simulink model "Test14Dof"  (R2024a)
settings: Solver=ode4  StartTime=0.0  StopTime=10.0  FixedStep=0.001  RelTol=1e-3
values from neighbouring files (symbols this model uses):
  EnvGrvty = 9.81    [Par.m]
  PlntBattChrgMax = 4.493    [Par.m]
  PlntBattNumCellSer = 96    [Par.m]
  PlntBattOpenCirctVolt = [3.17242 3.17242 3.17242 3.17242 3.17242 3.17242 3.17242;3.18272 3.18272 3.18272 3.18272 3.18272 3.18272 3.18272;3.19302 3.19302 3.19302 3.19302 3.19302 3.19302 3.19302;3.20331 3.20331 3.20331 3.20331 3.20331 3.20331 3.20331;3.21361 3.21361 3.21361 3.21361 3.21361 3.21361 3.21361;3.22391 3.22391 3.22391 3.22391 3.22391 3.22391 3.22391;3.23421 3.23421 3.23421 3.23421 3.23421 3.23421 3.23421;3.24451 ...(+5187 chars)    [Par.m]
  PlntBattSocInit = 0.6    [Par.m]
  PlntBattTempBpt = [-40 -30 -20 0 23 45 60]    [Par.m]
  PlntBattTempInitDegC = 25    [Par.m]
  PlntBattVoltSocBpt = [0 0.01 0.02 0.03 0.04 0.05 0.06 0.07 0.08 0.09 0.1 0.11 0.12 0.13 0.14 0.15 0.16 0.17 0.18 0.19 0.2 0.21 0.22 0.23 0.24 0.25 0.26 0.27 0.28 0.29 0.3 0.31 0.32 0.33 0.34 0.35 0.36 0.37 0.38 0.39 0.4 0.41 0.42 0.43 0.44 0.45 0.46 0.47 0.48 0.49 0.5 0.51 0.52 0.53 0.54 0.55 0.56 0.57 0.58 0.59 0.6 0.61 0.62 0.63 0.64 0.65 0.66 0.67 0.68 0.69 0.7 0.71 0.72 0.73 0.74 0.75 0.76 0.77 0.78 0.79 0.8 0.81  ...(+91 chars)    [Par.m]
  PlntDCDCVoltInit = 650    [Par.m]
  PlntDriveshftDamp = 100    [Par.m]
  PlntDriveshftStiff = 500    [Par.m]
  PlntEM1RotDamp = 0.001    [Par.m]
  PlntEM1RotInertia = 0.01    [Par.m]
  PlntEM2RotDamp = 0.001    [Par.m]
  PlntEM2RotInertia = 0.01    [Par.m]
  PlntEM3RotDamp = 0.001    [Par.m]
  PlntEM3RotInertia = 0.01    [Par.m]
  PlntEM4RotDamp = 0.001    [Par.m]
  PlntEM4RotInertia = 0.01    [Par.m]
  PlntEMWhlGearRatioFL = 11.04    [Par.m]
  PlntEMWhlGearRatioFR = 11.04    [Par.m]
  PlntEMWhlGearRatioRL = 11.04    [Par.m]
  PlntEMWhlGearRatioRR = 11.04    [Par.m]
  PlntSteerGearRatio = 52.025    [Par.m]
  PlntVehCGHgtAxl = 0.375    [Par.m]
  PlntVehDstCGFrntAxl = 1.61    [Par.m]
  PlntVehDstCGRearAxl = 1.39    [Par.m]
  PlntVehFrntUnsprgMass = 100    [Par.m]
  PlntVehInitLatPos = 0    [Par.m]
  PlntVehInitLatVel = 0    [Par.m]
  PlntVehInitLongPos = 0    [Par.m]
  PlntVehInitLongVel = 0    [Par.m]
  PlntVehInitPitchAng = 0    [Par.m]
  PlntVehInitPitchRate = 0    [Par.m]
  PlntVehInitRollAng = 0    [Par.m]
  PlntVehInitRollRate = 0    [Par.m]
  PlntVehInitVertPos = 0    [Par.m]
  PlntVehInitVertVel = 0    [Par.m]
  PlntVehInitYawAng = 0    [Par.m]
  PlntVehInitYawRate = 0    [Par.m]
  PlntVehMass = 2497    [Par.m]
  PlntVehPitchMomentInertia = 1922.7    [Par.m]
  PlntVehRearUnsprgMass = 100    [Par.m]
  PlntVehRollMomentInertia = 432.33333333333331    (= 432.333333333)    [Par.m]
  PlntVehTrckWdth = [1.685,1.685]    [Par.m]
  PlntVehYawMomentInertia = 2066    [Par.m]
  PlntWhlNumFrnt = 2    [Par.m]
  PlntWhlNumRear = 2    [Par.m]
  PlntWhlPrsFrnt = 220000    [Par.m]
  PlntWhlPrsRear = 220000    [Par.m]
undefined symbols (not defined in the file or in its folder): BdyFrm, InertFrm, PlntTrnsfrCaseAxlSpdLock, PlntTrnsfrCaseTrqSplitRatio
libraries: autolibsharedcoupling x12, autolibsharedcommon x12, autolibutils x10, autolibmappedmotor x4, autolibcoupling x4, matrix_library x4, vehdynlibsuspension x2, vehdynlibtire x2, vehdynlibtirecommon x2, vehdynlibsteering x2, shared6dof x2, autolibdatasheetbattery x1
(part 2 of 7)

== system Test14Dof/Subsystem/Vehicle 14 DoF model/Electric Machines/Subsystem1 ==
  EMTrqCmd : Inport
  EMSpd : Inport  Port=2
  BusVolt : Inport  Port=3
  Mapped Motor : autolibmappedmotor/Mapped Motor  port_config=Speed  param_by=Tabulated torque-speed envelope  w_t=PlntEM1Spd  T_t=PlntEM1Trq  torque_max=0.1  power_max=30  Tc=PlntEM1TimeCnst  param_loss=Tabulated efficiency data  eff=100  w_eff=375  T_eff=0.08  Piron=0  Pbase=0  w_eff_bp=PlntEM1SpdEff  T_eff_bp=PlntEM1TrqEff  Temp_eff_bp=Temp_eff_bp  losses_table=PlntEM1TrqLossTbl  losses_table_3d=losses_table_3d  efficiency_table=PlntEM1EffTbl  efficiency_table_3d=efficiency_table_3d  J=5e-6  b=1e-5  omega_o=0  T_t_extended=[125.931348721462 137.379653150686 151.117618465755 167.90846496195 188.897023082193 215.882312093935 251.862697442924 302.235236931509 377.794046164387 450 450 450 450 450 450 450 450 450 377.794046164387 302.235236931509 251.862697442924 215.882312093935 188.897023082193 167.90846496195 151.117618465755 137.379653150686 125.931348721462]  w_t_extended=[-1675.51608191456 -1535.88974175501 -1396.26340159546 -1256.63706143592 -1117.01072127637 -977.384381116825 -837.758040957278 -698.131700797732 -558.505360638185 -468.888888888889 -418.879020478639 -279.252680319093 -139.626340159546 0 139.626340159546 279.252680319093 418.879020478639 468.888888888889 558.505360638185 698.131700797732 837.758040957278 977.384381116825 1117.01072127637 1256.63706143592 1396.26340159546 1535.88974175501 1675.51608191456]  KLossIron=0  KLossCopper=0  x_w_eff_vec=[-1675.51608191456 -1535.88974175501 -1396.26340159546 -1256.63706143592 -1117.01072127637 -977.384381116825 -837.758040957278 -698.131700797732 -558.505360638185 -468.888888888889 -418.879020478639 -279.252680319093 -139.626340159546 0 139.626340159546 279.252680319093 418.879020478639 468.888888888889 558.505360638185 698.131700797732 837.758040957278 977.384381116825 1117.01072127637 1256.63706143592 1396.26340159546 1535.88974175501 1675.51608191456]  x_T_eff_vec=[-450 -405 -360 -315 -270 -225 -180 -135 -90 -45 0 45 90 135 180 225 270 315 360 405 450]  x_tmp_eff_vec=[233.15 293.15 373.15]  x_losses_mat=[56751.351161622 51076.2160454598 45401.0809292976 39725.9458131354 34050.8106969732 28375.675580811 22700.5404646488 17025.4053484866 14913.9343555032 12274.1294372811 0 10555.7513160617 13571.6802635079 15833.6269740925 21111.5026321234 26389.3782901542 31667.2539481851 36945.1296062159 42223.0052642468 47500.8809222776 52778.7565803085;52022.0718981535 46819.8647083382 41617.6575185228 36415.4503287075 31213.2431388921 26011.0359490768 20808.8287592614 15606.6215694461 12020.0066746044 11251.2853175076 0 9676.10537305656 11058.4061406361 14514.1580595848 19352.2107461131 24190.2634326414 29028.3161191697 33866.3688056979 38704.4214922262 43542.4741787545 48380.5268652828;47292.792634685 42563.5133712165 37834.234107748 33104.9548442795 28375.675580811 23646.3963173425 18917.117053874 14187.8377904055 10927.2787950949 10228.4411977342 0 8796.45943005142 10053.0964914873 13194.6891450771 17592.9188601028 21991.1485751285 26389.3782901542 30787.60800518 35185.8377202057 39584.0674352314 43982.2971502571;42563.5133712165 38307.1620340949 34050.8106969732 29794.4593598516 25538.1080227299 21281.7566856083 17025.4053484866 12769.054011365 11185.4507666274 9205.59707796079 0 7916.81348704628 10178.7601976309 11875.2202305694 15833.6269740925 19792.0337176157 23750.4404611388 27708.847204662 31667.2539481851 35625.6606917082 39584.0674352314;37834.234107748 34050.8106969732 30267.3872861984 26483.9638754236 22700.5404646488 18917.117053874 15133.6936430992 11350.2702323244 9942.62290366878 8182.75295818737 0 7037.16754404114 9047.7868423386 10555.7513160617 14074.3350880823 17592.9188601028 21111.5026321234 24630.086404144 28148.6701761645 31667.2539481851 35185.8377202057;33104.9548442795 29794.4593598516 26483.9638754236 23173.4683909957 19862.9729065677 16552.4774221398 15298.1903131329 11473.6427348497 9773.84381116825 8377.58040957278 0 7037.16754404114 8796.45943005142 10555.7513160617 14074.3350880823 15393.80400259 18472.564803108 21551.325603626 24630.086404144 27708.847204662 30787.60800518;28375.675580811 25538.1080227299 22700.5404646488 19862.9729065677 17025.4053484866 16390.9181926424 14913.9343555032 11185.4507666274 10281.575957203 8275.41479482189 0 6785.84013175395 9047.7868423386 10178.7601976309 13571.6802635079 15079.644737231 15833.6269740925 18472.564803108 21111.5026321234 23750.4404611388 26389.3782901542;31070.6965739649 27963.6269165685 21854.5575901899 19122.7378914161 16390.9181926424 15535.3482869825 12428.278629586 10471.975511966 8567.97996433581 6896.17899568491 0 5654.86677646163 7539.8223686155 9424.77796076938 11309.7335529233 14137.1669411541 15079.644737231 17592.9188601028 20106.1929829747 25446.9004940773 28274.3338823081;34271.9198573432 30844.7278716089 27417.5358858746 19547.6876223365 16755.1608191456 13962.6340159546 11170.1072127637 10281.575957203 8182.75295818737 6283.18530717959 0 5026.54824574367 7037.16754404114 9047.78684233861 10053.0964914873 12566.3706143592 15079.644737231 17592.9188601028 24127.4315795696 27143.3605270158 30159.289474462;34348.8372093023 30913.9534883721 27479.0697674419 20140.9090909091 17263.6363636364 14386.3636363636 11509.0909090909 8631.81818181819 6869.76744186047 5275 0 4220 5908 7596 10128 12660 15192 17724 23632 26586 29540;35903.9160410262 32313.5244369236 24548.2588745621 21479.7265152418 15422.3639358044 12851.9699465037 10281.575957203 9205.59707796079 6137.06471864053 4712.38898038469 0 3769.91118430775 5277.87565803085 7916.81348704628 9047.7868423386 11309.7335529233 13571.6802635079 18472.564803108 21111.5026321234 27143.3605270158 30159.289474462;27584.7159827396 24826.2443844657 19148.7552218806 16755.1608191456 12274.1294372811 10228.4411977342 8182.75295818737 6137.06471864053 4787.18880547016 3544.36094251156 0 2764.60153515902 4021.23859659494 5277.87565803085 7037.16754404114 8796.45943005142 10555.7513160617 14074.3350880823 16084.9543863797 20357.5203952619 22619.4671058465;26927.9370307696 19868.4508362165 15873.3102497169 ...(+4614 chars)]  x_losses_mat_3d=cat(3,[2 2 2 2 2 2 2 2 2 2 2 2 2 2 2 2 2 2 2 2 2;2 2 2 2 2 2 2 2 2 2 2 2 2 2 2 2 2 2 2 2 2;2 2 2 2 2 2 2 2 2 2 2 2 2 2 2 2 2 2 2 2 2;2 2 2 2 2 2 2 2 2 2 2 2 2 2 2 2 2 2 2 2 2;2 2 2 2 2 2 2 2 2 2 2 2 2 2 2 2 2 2 2 2 2;2 2 2 2 2 2 2 2 2 2 2 2 2 2 2 2 2 2 2 2 2;2 2 2 2 2 2 2 2 2 2 2 2 2 2 2 2 2 2 2 2 2;2 2 2 2 2 2 2 2 2 2 2 2 2 2 2 2 2 2 2 2 2;2 2 2 2 2 2 2 2 2 2 2 2 2 2 2 2 2 2 2 2 2;2 2 2 2 2 2 2 2 2 2 2 2 2 2 2 2 2 2 2 2 2;2 2 2 2 2 2 2 2 2 2 2 2 2 2 2 2 2 2 2 2 2;2 2 2 2 2 2 2 2 2 2 2 2 2 2 2 2 2 2 2 2 2;2 2 2 2 2 2 2 2 2 2 2 2 2 2 2 2 2 2 2 2 2;2 2 2 2 2 2 2 2 2 2 2 2 2 2 2 2 2 2 2 2 2;2 2 2 2 2 2 2 2 2 2 2 2 2 2 2 2 2 2 2 2 2;2 2 2 2 2 2 2 2 2 2 2 2 2 2 2 2 2 2 2 2 2;2 2 2 2 2 2 2 2 2 2 2 2 2 2 2 2 2 2 2 2 2;2 2 2 2 2 2 2 2 2 2 2 2 2 2 2 2 2 2 2 2 2;2 2 2 2 2 2 2 2 2 2 2 2 2 2 2 2 2 2 2 2 2;2 2 2 2 2 2 2 2 2 2 2 2 2 2 2 2 2 2 2 2 2;2 2 2 2 2 2 2 2 2 2 2 2 2 2 2 2 2 2 2 2 2;2 2 2 2 2 2 2 2 2 2 2 2 2 2 2 2 2 2 2 2 2;2 2 2 2 2 2 2 2 2 2 2 2 2 2 2 2 2 2 2 2 2;2 2 2 2 2 2 2 2 2 2 2 2 2 2 2 2 2 2 2 2 2;2 2 2 2 2 2 2 2 2 2 2 2 2 2 2 2 2 2 2 2 2;2 2 2 2 2 2 2 2 2 2 2 2 2 2 2 2 2 2 2 2 2;2 2 2 2 2 2 2 2 2 2 2 2 2 2 2 2 2 2 2 2 2],[1.5 1.5 1.5 1.5 1.5 1.5 1.5 1.5 1.5 1.5 1.5 1.5 1.5 1.5 1.5 1.5 1.5 1.5 1.5 1.5 1.5;1.5 1.5 1.5 1.5 1.5 1.5 1.5 1.5 1.5 1.5 1.5 1.5 1.5 1.5 1.5 1.5 1.5 1.5 1.5 1.5 1.5;1.5 1.5 1.5 1.5 1.5 1.5 1.5 1.5 1.5 1.5 1.5 1.5 1.5 1.5 1.5 1.5 1.5 1.5 1.5 1.5 1.5;1.5 1.5 1.5 1.5 1.5 1.5 1.5 1.5 1.5 1.5 1.5 1.5 1.5 1.5 1.5 1.5 1.5 1.5 1.5 1.5 1.5;1.5 1.5 1.5 1.5 1.5 1.5 1.5 1.5 1.5 1.5 1.5 1.5 1.5 1.5 1.5 1.5 1.5 1.5 1.5 1.5 1.5;1.5 1.5 1.5 1.5 1.5 1.5 1.5 1.5 1.5 1.5 1.5 1.5 1.5 1.5 1.5 1.5 1.5 1.5 1.5 1.5 1.5;1.5 1.5 1.5 1.5 1.5 1.5 1.5 1.5 1.5 1.5 1.5 1.5 1.5 1.5 1.5 1.5 1.5 1.5 1.5 1.5 1.5;1.5 1.5 1.5 1.5 1.5 1.5 1.5 1.5 1.5 1.5 1.5 1.5 1.5 1.5 1.5 1.5 1.5 1.5 1.5 1.5 1.5;1.5 1.5 1.5 1.5 1.5 1.5 1.5 1.5 1.5 1.5 1.5 1.5 1.5 1.5 1.5 1.5 1.5 1.5 1.5 1.5 1.5;1.5 1.5 1.5 1.5 1.5 1.5 1.5 1.5 1.5 1.5 1.5 1.5 1.5 1.5 1.5 1.5 1.5 1.5 1.5 1.5 1.5;1.5 1.5 1.5 1.5 1.5 1.5 1.5 1.5 1.5 1.5 1.5 1.5 1.5 1.5 1.5 1.5 1.5 1.5 1.5 1.5 1.5;1.5 1.5 1.5 1.5 1.5 1.5 1.5 1.5 1.5 1.5 1.5 1.5 1.5 1.5 1.5 1.5 1.5 1.5 1.5 1.5 1.5;1.5 1.5 1.5 1.5 1.5 1.5 1.5 1.5 1.5 1.5 1.5 1.5 1.5 1.5 1.5 1.5 1.5 1.5 1.5 1.5 1.5;1.5 1.5 1.5 1.5 1.5 1.5 1.5 1.5 1.5 1.5 1.5 1.5 1.5 1.5 1.5 1.5 1.5 1.5 1.5 1.5 1.5;1.5 1.5 1.5 1.5 1.5 1.5 1.5 1.5 1.5 1.5 1.5 1.5 1.5 1.5 1.5 1.5 1.5 1.5 1.5 1.5 1.5;1.5 1.5 1.5 1.5 1.5 1.5 1.5 1.5 1.5 1.5 1.5 1.5 1.5 1.5 1.5 1.5 1.5 1.5 1.5 1.5 1.5;1.5 1.5 1.5 1.5 1.5 1.5 1.5 1.5 1.5 1.5 1.5 1.5 1.5 1.5 1.5 1.5 1.5 1.5 1.5 1.5 1.5;1.5 1.5 1.5 1.5 1.5 1.5 1.5 1.5 1.5 1.5 1.5 1.5 1.5 1.5 1.5 1.5 1.5 1.5 1.5 1.5 1.5;1.5 1.5 1.5 1.5 1.5 1.5 1.5 1.5 1.5 1.5 1.5 1.5 1.5 1.5 1.5 1.5 1.5 1.5 1.5 1.5 1.5;1.5 1.5 1.5 1.5 1.5 1.5 1.5 1.5 1.5 1.5 1.5 1.5 1.5 1.5 1.5 1.5 1.5 1.5 1.5 1.5 1.5;1.5 1.5 1.5 1.5 1.5 1.5 1.5 1.5 1.5 1.5 1.5 1.5 1.5 1.5 1.5 1.5 1.5 1.5 1.5 1.5 1.5;1.5 1.5 1.5 1.5 1.5 1.5 1.5 1.5 1.5 1.5 1.5 1.5 1.5 1.5 1.5 1.5 1.5 1.5 1.5 1.5 1.5;1.5 1.5 1.5 1.5 1.5 1.5 1.5 1.5 1.5 1.5 1.5 1.5 1.5 1.5 1.5 1.5 1.5 1.5 1.5 1.5 1.5;1.5 1.5 1.5 1.5 1.5 1.5 1.5 1.5 1.5 1.5 1.5 1.5 1.5 1.5 1.5 1.5 1.5 1.5 1.5 1.5 1.5;1.5 1.5 1.5 1.5 1.5 1.5 1.5 1.5 1.5 1.5 1.5 1.5 1.5 1.5 1.5 1.5 1.5 1.5 1.5 1.5 1.5;1.5 1.5 1.5 1.5 1.5 1.5 1.5 1.5 1.5 1.5 1.5 1.5 1.5 1.5 1.5 1.5 1.5 1.5 1.5 1.5 1.5;1.5 1.5 1.5 1.5 1.5 1.5 1.5 1.5 1.5 1.5 1.5 1.5 1.5 1.5 1.5 1.5 1.5 1.5 1.5 1.5 1.5],[1.9 1.9 1.9 1.9 1.9 1.9 1.9 1.9 1.9 1.9 1.9 1.9 1.9 1.9 1.9 1.9 1.9 1.9 1.9 1.9 1.9;1.9 1.9 1.9 1.9 1.9 1.9 1.9 1.9 1.9 1.9 1.9 1.9 1.9 1.9 1.9 1.9 1.9 1.9 1.9 1.9 1.9;1.9 1.9 1.9 1.9 1.9 1.9 1.9 1.9 1.9 1.9 1.9 1.9 1.9 1.9 1.9 1.9 1.9 1.9 1.9 1.9 1.9;1.9 1.9 1.9 1.9 1.9 1.9 1.9 1.9 1.9 1.9 1.9 1.9 1.9 1.9 1.9 1.9 1.9 1.9 1.9 1.9 1.9;1.9 1.9 1.9 1.9 1.9 1.9 1.9 1.9 1.9 1.9 1.9 1.9 1.9 1.9 1.9 1.9 1.9 1.9 1.9 1.9 1.9;1.9 1.9 1.9 1.9 1.9 1.9 1.9 1.9 1.9 1.9 1.9 1.9 1.9 1.9 1.9 1.9 1.9 1.9 1.9 1.9 1.9;1.9 1.9 1.9 1.9 1.9 1.9 1.9 1.9 1.9 1.9 1.9 1.9 1.9 1.9 1.9 1.9 1.9 1.9 1.9 1.9 1.9 ...(+1680 chars)])  CalLossMapData={'BaseCageProjectFileName','';'BaseMbcProjectFileName','';'TaskName','Calibrate Motor Loss Map';'ChildTasks',{{'DataName','';'TaskName','Import Loss Data'},{'TaskName','Generate Response Models'},{'TaskName','Generate Calibration'},{'TaskName','Update Block Parameters'}}}  CalLossWithTempMapData={}  aMode=6  RefBlkName='autolibmappedmotor/Mapped Motor'
  EMTrq : Outport  VectorParamsAs1DForOutWhenUnconnected=off
  EMCurr : Outport  Port=2  VectorParamsAs1DForOutWhenUnconnected=off
  Info : Outport  Port=3
  wires:
  BusVolt/1 -> Mapped Motor/1
  EMSpd/1 -> Mapped Motor/2
  EMTrqCmd/1 -> Mapped Motor/3
  Mapped Motor/1 -> Info/1
  Mapped Motor/2 -> EMCurr/1
  Mapped Motor/3 -> EMTrq/1

== system Test14Dof/Subsystem/Vehicle 14 DoF model/Electric Machines/Subsystem2 ==
  EMTrqCmd : Inport
  EMSpd : Inport  Port=2
  BusVolt : Inport  Port=3
  Mapped Motor : autolibmappedmotor/Mapped Motor  port_config=Speed  param_by=Tabulated torque-speed envelope  w_t=PlntEM1Spd  T_t=PlntEM1Trq  torque_max=0.1  power_max=30  Tc=PlntEM1TimeCnst  param_loss=Tabulated efficiency data  eff=100  w_eff=375  T_eff=0.08  Piron=0  Pbase=0  w_eff_bp=PlntEM1SpdEff  T_eff_bp=PlntEM1TrqEff  Temp_eff_bp=Temp_eff_bp  losses_table=PlntEM1TrqLossTbl  losses_table_3d=losses_table_3d  efficiency_table=PlntEM1EffTbl  efficiency_table_3d=efficiency_table_3d  J=5e-6  b=1e-5  omega_o=0  T_t_extended=[125.931348721462 137.379653150686 151.117618465755 167.90846496195 188.897023082193 215.882312093935 251.862697442924 302.235236931509 377.794046164387 450 450 450 450 450 450 450 450 450 377.794046164387 302.235236931509 251.862697442924 215.882312093935 188.897023082193 167.90846496195 151.117618465755 137.379653150686 125.931348721462]  w_t_extended=[-1675.51608191456 -1535.88974175501 -1396.26340159546 -1256.63706143592 -1117.01072127637 -977.384381116825 -837.758040957278 -698.131700797732 -558.505360638185 -468.888888888889 -418.879020478639 -279.252680319093 -139.626340159546 0 139.626340159546 279.252680319093 418.879020478639 468.888888888889 558.505360638185 698.131700797732 837.758040957278 977.384381116825 1117.01072127637 1256.63706143592 1396.26340159546 1535.88974175501 1675.51608191456]  KLossIron=0  KLossCopper=0  x_w_eff_vec=[-1675.51608191456 -1535.88974175501 -1396.26340159546 -1256.63706143592 -1117.01072127637 -977.384381116825 -837.758040957278 -698.131700797732 -558.505360638185 -468.888888888889 -418.879020478639 -279.252680319093 -139.626340159546 0 139.626340159546 279.252680319093 418.879020478639 468.888888888889 558.505360638185 698.131700797732 837.758040957278 977.384381116825 1117.01072127637 1256.63706143592 1396.26340159546 1535.88974175501 1675.51608191456]  x_T_eff_vec=[-450 -405 -360 -315 -270 -225 -180 -135 -90 -45 0 45 90 135 180 225 270 315 360 405 450]  x_tmp_eff_vec=[233.15 293.15 373.15]  x_losses_mat=[56751.351161622 51076.2160454598 45401.0809292976 39725.9458131354 34050.8106969732 28375.675580811 22700.5404646488 17025.4053484866 14913.9343555032 12274.1294372811 0 10555.7513160617 13571.6802635079 15833.6269740925 21111.5026321234 26389.3782901542 31667.2539481851 36945.1296062159 42223.0052642468 47500.8809222776 52778.7565803085;52022.0718981535 46819.8647083382 41617.6575185228 36415.4503287075 31213.2431388921 26011.0359490768 20808.8287592614 15606.6215694461 12020.0066746044 11251.2853175076 0 9676.10537305656 11058.4061406361 14514.1580595848 19352.2107461131 24190.2634326414 29028.3161191697 33866.3688056979 38704.4214922262 43542.4741787545 48380.5268652828;47292.792634685 42563.5133712165 37834.234107748 33104.9548442795 28375.675580811 23646.3963173425 18917.117053874 14187.8377904055 10927.2787950949 10228.4411977342 0 8796.45943005142 10053.0964914873 13194.6891450771 17592.9188601028 21991.1485751285 26389.3782901542 30787.60800518 35185.8377202057 39584.0674352314 43982.2971502571;42563.5133712165 38307.1620340949 34050.8106969732 29794.4593598516 25538.1080227299 21281.7566856083 17025.4053484866 12769.054011365 11185.4507666274 9205.59707796079 0 7916.81348704628 10178.7601976309 11875.2202305694 15833.6269740925 19792.0337176157 23750.4404611388 27708.847204662 31667.2539481851 35625.6606917082 39584.0674352314;37834.234107748 34050.8106969732 30267.3872861984 26483.9638754236 22700.5404646488 18917.117053874 15133.6936430992 11350.2702323244 9942.62290366878 8182.75295818737 0 7037.16754404114 9047.7868423386 10555.7513160617 14074.3350880823 17592.9188601028 21111.5026321234 24630.086404144 28148.6701761645 31667.2539481851 35185.8377202057;33104.9548442795 29794.4593598516 26483.9638754236 23173.4683909957 19862.9729065677 16552.4774221398 15298.1903131329 11473.6427348497 9773.84381116825 8377.58040957278 0 7037.16754404114 8796.45943005142 10555.7513160617 14074.3350880823 15393.80400259 18472.564803108 21551.325603626 24630.086404144 27708.847204662 30787.60800518;28375.675580811 25538.1080227299 22700.5404646488 19862.9729065677 17025.4053484866 16390.9181926424 14913.9343555032 11185.4507666274 10281.575957203 8275.41479482189 0 6785.84013175395 9047.7868423386 10178.7601976309 13571.6802635079 15079.644737231 15833.6269740925 18472.564803108 21111.5026321234 23750.4404611388 26389.3782901542;31070.6965739649 27963.6269165685 21854.5575901899 19122.7378914161 16390.9181926424 15535.3482869825 12428.278629586 10471.975511966 8567.97996433581 6896.17899568491 0 5654.86677646163 7539.8223686155 9424.77796076938 11309.7335529233 14137.1669411541 15079.644737231 17592.9188601028 20106.1929829747 25446.9004940773 28274.3338823081;34271.9198573432 30844.7278716089 27417.5358858746 19547.6876223365 16755.1608191456 13962.6340159546 11170.1072127637 10281.575957203 8182.75295818737 6283.18530717959 0 5026.54824574367 7037.16754404114 9047.78684233861 10053.0964914873 12566.3706143592 15079.644737231 17592.9188601028 24127.4315795696 27143.3605270158 30159.289474462;34348.8372093023 30913.9534883721 27479.0697674419 20140.9090909091 17263.6363636364 14386.3636363636 11509.0909090909 8631.81818181819 6869.76744186047 5275 0 4220 5908 7596 10128 12660 15192 17724 23632 26586 29540;35903.9160410262 32313.5244369236 24548.2588745621 21479.7265152418 15422.3639358044 12851.9699465037 10281.575957203 9205.59707796079 6137.06471864053 4712.38898038469 0 3769.91118430775 5277.87565803085 7916.81348704628 9047.7868423386 11309.7335529233 13571.6802635079 18472.564803108 21111.5026321234 27143.3605270158 30159.289474462;27584.7159827396 24826.2443844657 19148.7552218806 16755.1608191456 12274.1294372811 10228.4411977342 8182.75295818737 6137.06471864053 4787.18880547016 3544.36094251156 0 2764.60153515902 4021.23859659494 5277.87565803085 7037.16754404114 8796.45943005142 10555.7513160617 14074.3350880823 16084.9543863797 20357.5203952619 22619.4671058465;26927.9370307696 19868.4508362165 15873.3102497169 ...(+4614 chars)]  x_losses_mat_3d=cat(3,[2 2 2 2 2 2 2 2 2 2 2 2 2 2 2 2 2 2 2 2 2;2 2 2 2 2 2 2 2 2 2 2 2 2 2 2 2 2 2 2 2 2;2 2 2 2 2 2 2 2 2 2 2 2 2 2 2 2 2 2 2 2 2;2 2 2 2 2 2 2 2 2 2 2 2 2 2 2 2 2 2 2 2 2;2 2 2 2 2 2 2 2 2 2 2 2 2 2 2 2 2 2 2 2 2;2 2 2 2 2 2 2 2 2 2 2 2 2 2 2 2 2 2 2 2 2;2 2 2 2 2 2 2 2 2 2 2 2 2 2 2 2 2 2 2 2 2;2 2 2 2 2 2 2 2 2 2 2 2 2 2 2 2 2 2 2 2 2;2 2 2 2 2 2 2 2 2 2 2 2 2 2 2 2 2 2 2 2 2;2 2 2 2 2 2 2 2 2 2 2 2 2 2 2 2 2 2 2 2 2;2 2 2 2 2 2 2 2 2 2 2 2 2 2 2 2 2 2 2 2 2;2 2 2 2 2 2 2 2 2 2 2 2 2 2 2 2 2 2 2 2 2;2 2 2 2 2 2 2 2 2 2 2 2 2 2 2 2 2 2 2 2 2;2 2 2 2 2 2 2 2 2 2 2 2 2 2 2 2 2 2 2 2 2;2 2 2 2 2 2 2 2 2 2 2 2 2 2 2 2 2 2 2 2 2;2 2 2 2 2 2 2 2 2 2 2 2 2 2 2 2 2 2 2 2 2;2 2 2 2 2 2 2 2 2 2 2 2 2 2 2 2 2 2 2 2 2;2 2 2 2 2 2 2 2 2 2 2 2 2 2 2 2 2 2 2 2 2;2 2 2 2 2 2 2 2 2 2 2 2 2 2 2 2 2 2 2 2 2;2 2 2 2 2 2 2 2 2 2 2 2 2 2 2 2 2 2 2 2 2;2 2 2 2 2 2 2 2 2 2 2 2 2 2 2 2 2 2 2 2 2;2 2 2 2 2 2 2 2 2 2 2 2 2 2 2 2 2 2 2 2 2;2 2 2 2 2 2 2 2 2 2 2 2 2 2 2 2 2 2 2 2 2;2 2 2 2 2 2 2 2 2 2 2 2 2 2 2 2 2 2 2 2 2;2 2 2 2 2 2 2 2 2 2 2 2 2 2 2 2 2 2 2 2 2;2 2 2 2 2 2 2 2 2 2 2 2 2 2 2 2 2 2 2 2 2;2 2 2 2 2 2 2 2 2 2 2 2 2 2 2 2 2 2 2 2 2],[1.5 1.5 1.5 1.5 1.5 1.5 1.5 1.5 1.5 1.5 1.5 1.5 1.5 1.5 1.5 1.5 1.5 1.5 1.5 1.5 1.5;1.5 1.5 1.5 1.5 1.5 1.5 1.5 1.5 1.5 1.5 1.5 1.5 1.5 1.5 1.5 1.5 1.5 1.5 1.5 1.5 1.5;1.5 1.5 1.5 1.5 1.5 1.5 1.5 1.5 1.5 1.5 1.5 1.5 1.5 1.5 1.5 1.5 1.5 1.5 1.5 1.5 1.5;1.5 1.5 1.5 1.5 1.5 1.5 1.5 1.5 1.5 1.5 1.5 1.5 1.5 1.5 1.5 1.5 1.5 1.5 1.5 1.5 1.5;1.5 1.5 1.5 1.5 1.5 1.5 1.5 1.5 1.5 1.5 1.5 1.5 1.5 1.5 1.5 1.5 1.5 1.5 1.5 1.5 1.5;1.5 1.5 1.5 1.5 1.5 1.5 1.5 1.5 1.5 1.5 1.5 1.5 1.5 1.5 1.5 1.5 1.5 1.5 1.5 1.5 1.5;1.5 1.5 1.5 1.5 1.5 1.5 1.5 1.5 1.5 1.5 1.5 1.5 1.5 1.5 1.5 1.5 1.5 1.5 1.5 1.5 1.5;1.5 1.5 1.5 1.5 1.5 1.5 1.5 1.5 1.5 1.5 1.5 1.5 1.5 1.5 1.5 1.5 1.5 1.5 1.5 1.5 1.5;1.5 1.5 1.5 1.5 1.5 1.5 1.5 1.5 1.5 1.5 1.5 1.5 1.5 1.5 1.5 1.5 1.5 1.5 1.5 1.5 1.5;1.5 1.5 1.5 1.5 1.5 1.5 1.5 1.5 1.5 1.5 1.5 1.5 1.5 1.5 1.5 1.5 1.5 1.5 1.5 1.5 1.5;1.5 1.5 1.5 1.5 1.5 1.5 1.5 1.5 1.5 1.5 1.5 1.5 1.5 1.5 1.5 1.5 1.5 1.5 1.5 1.5 1.5;1.5 1.5 1.5 1.5 1.5 1.5 1.5 1.5 1.5 1.5 1.5 1.5 1.5 1.5 1.5 1.5 1.5 1.5 1.5 1.5 1.5;1.5 1.5 1.5 1.5 1.5 1.5 1.5 1.5 1.5 1.5 1.5 1.5 1.5 1.5 1.5 1.5 1.5 1.5 1.5 1.5 1.5;1.5 1.5 1.5 1.5 1.5 1.5 1.5 1.5 1.5 1.5 1.5 1.5 1.5 1.5 1.5 1.5 1.5 1.5 1.5 1.5 1.5;1.5 1.5 1.5 1.5 1.5 1.5 1.5 1.5 1.5 1.5 1.5 1.5 1.5 1.5 1.5 1.5 1.5 1.5 1.5 1.5 1.5;1.5 1.5 1.5 1.5 1.5 1.5 1.5 1.5 1.5 1.5 1.5 1.5 1.5 1.5 1.5 1.5 1.5 1.5 1.5 1.5 1.5;1.5 1.5 1.5 1.5 1.5 1.5 1.5 1.5 1.5 1.5 1.5 1.5 1.5 1.5 1.5 1.5 1.5 1.5 1.5 1.5 1.5;1.5 1.5 1.5 1.5 1.5 1.5 1.5 1.5 1.5 1.5 1.5 1.5 1.5 1.5 1.5 1.5 1.5 1.5 1.5 1.5 1.5;1.5 1.5 1.5 1.5 1.5 1.5 1.5 1.5 1.5 1.5 1.5 1.5 1.5 1.5 1.5 1.5 1.5 1.5 1.5 1.5 1.5;1.5 1.5 1.5 1.5 1.5 1.5 1.5 1.5 1.5 1.5 1.5 1.5 1.5 1.5 1.5 1.5 1.5 1.5 1.5 1.5 1.5;1.5 1.5 1.5 1.5 1.5 1.5 1.5 1.5 1.5 1.5 1.5 1.5 1.5 1.5 1.5 1.5 1.5 1.5 1.5 1.5 1.5;1.5 1.5 1.5 1.5 1.5 1.5 1.5 1.5 1.5 1.5 1.5 1.5 1.5 1.5 1.5 1.5 1.5 1.5 1.5 1.5 1.5;1.5 1.5 1.5 1.5 1.5 1.5 1.5 1.5 1.5 1.5 1.5 1.5 1.5 1.5 1.5 1.5 1.5 1.5 1.5 1.5 1.5;1.5 1.5 1.5 1.5 1.5 1.5 1.5 1.5 1.5 1.5 1.5 1.5 1.5 1.5 1.5 1.5 1.5 1.5 1.5 1.5 1.5;1.5 1.5 1.5 1.5 1.5 1.5 1.5 1.5 1.5 1.5 1.5 1.5 1.5 1.5 1.5 1.5 1.5 1.5 1.5 1.5 1.5;1.5 1.5 1.5 1.5 1.5 1.5 1.5 1.5 1.5 1.5 1.5 1.5 1.5 1.5 1.5 1.5 1.5 1.5 1.5 1.5 1.5;1.5 1.5 1.5 1.5 1.5 1.5 1.5 1.5 1.5 1.5 1.5 1.5 1.5 1.5 1.5 1.5 1.5 1.5 1.5 1.5 1.5],[1.9 1.9 1.9 1.9 1.9 1.9 1.9 1.9 1.9 1.9 1.9 1.9 1.9 1.9 1.9 1.9 1.9 1.9 1.9 1.9 1.9;1.9 1.9 1.9 1.9 1.9 1.9 1.9 1.9 1.9 1.9 1.9 1.9 1.9 1.9 1.9 1.9 1.9 1.9 1.9 1.9 1.9;1.9 1.9 1.9 1.9 1.9 1.9 1.9 1.9 1.9 1.9 1.9 1.9 1.9 1.9 1.9 1.9 1.9 1.9 1.9 1.9 1.9;1.9 1.9 1.9 1.9 1.9 1.9 1.9 1.9 1.9 1.9 1.9 1.9 1.9 1.9 1.9 1.9 1.9 1.9 1.9 1.9 1.9;1.9 1.9 1.9 1.9 1.9 1.9 1.9 1.9 1.9 1.9 1.9 1.9 1.9 1.9 1.9 1.9 1.9 1.9 1.9 1.9 1.9;1.9 1.9 1.9 1.9 1.9 1.9 1.9 1.9 1.9 1.9 1.9 1.9 1.9 1.9 1.9 1.9 1.9 1.9 1.9 1.9 1.9;1.9 1.9 1.9 1.9 1.9 1.9 1.9 1.9 1.9 1.9 1.9 1.9 1.9 1.9 1.9 1.9 1.9 1.9 1.9 1.9 1.9 ...(+1680 chars)])  CalLossMapData={'BaseCageProjectFileName','';'BaseMbcProjectFileName','';'TaskName','Calibrate Motor Loss Map';'ChildTasks',{{'DataName','';'TaskName','Import Loss Data'},{'TaskName','Generate Response Models'},{'TaskName','Generate Calibration'},{'TaskName','Update Block Parameters'}}}  CalLossWithTempMapData={}  aMode=6  RefBlkName='autolibmappedmotor/Mapped Motor'
  EMTrq : Outport  VectorParamsAs1DForOutWhenUnconnected=off
  EMCurr : Outport  Port=2  VectorParamsAs1DForOutWhenUnconnected=off
  Info : Outport  Port=3
  wires:
  BusVolt/1 -> Mapped Motor/1
  EMSpd/1 -> Mapped Motor/2
  EMTrqCmd/1 -> Mapped Motor/3
  Mapped Motor/1 -> Info/1
  Mapped Motor/2 -> EMCurr/1
  Mapped Motor/3 -> EMTrq/1
